simulink model "mpc_02_sim"  (R2020b)
settings: Solver=ode4  StartTime=0.0  StopTime=t_sim  FixedStep=T  RelTol=1e-3
values from neighbouring files (symbols this model uses):
  v_des = 1    [main_mpc_02.m]
  x0 = [1; 1; pi/2]    [main_mpc_02.m]
undefined symbols (not defined in the file or in its folder): mpc_ctrl_param
settings Model: Creator=vince  LastModifiedBy=vince
settings DataIOCC: ReturnWorkspaceOutputs=off

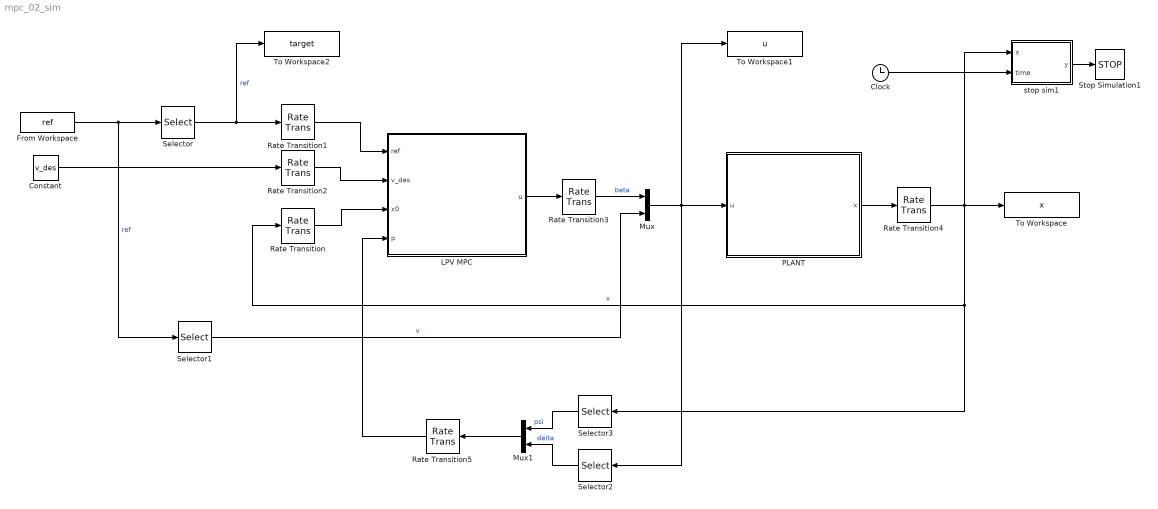
== system mpc_02_sim ==
  Clock : Clock
  Constant : Constant  Value=v_des
  From Workspace : FromWorkspace  VariableName=ref
  LPV MPC : Subsystem
  Mux : Mux  Inputs=2
  Mux1 : Mux  Inputs=2
  PLANT : Subsystem
  Rate Transition{,1..2,5} (4 alike) : RateTransition  OutPortSampleTime=mpc_ctrl_param.Ts
  Rate Transition3 : RateTransition  OutPortSampleTime=T
  Rate Transition4 : RateTransition  OutPortSampleTime=T
  Selector : Selector  InputPortWidth=4  IndexOptions=Index vector (dialog)  Indices=1:2  OutputSizes=1
  Selector1 : Selector  InputPortWidth=4  IndexOptions=Index vector (dialog)  Indices=4  OutputSizes=1
  Selector2 : Selector  InputPortWidth=2  IndexOptions=Index vector (dialog)  Indices=1  OutputSizes=1
  Selector3 : Selector  InputPortWidth=3  IndexOptions=Index vector (dialog)  Indices=3  OutputSizes=1
  Stop Simulation1 : Stop
  To Workspace : ToWorkspace  VariableName=x  SaveFormat=Timeseries  SampleTime=-1
  To Workspace1 : ToWorkspace  VariableName=u  SaveFormat=Timeseries  SampleTime=-1
  To Workspace2 : ToWorkspace  VariableName=target  SaveFormat=Timeseries  SampleTime=-1
  stop sim1 : MATLAB Function  TreatAsAtomicUnit=on
  wires:
  PLANT/1(x) -> Rate Transition4/1
  LPV MPC/1(u) -> Rate Transition3/1
  Rate Transition1/1 -> LPV MPC/1(ref)
  Rate Transition/1 -> LPV MPC/3(x0)
  Mux/1 -> To Workspace1/1, PLANT/1(u), Selector2/1
  From Workspace/1 -> Selector1/1, Selector/1  "ref"
  Selector/1 -> To Workspace2/1, Rate Transition1/1  "ref"
  Rate Transition3/1 -> Mux/1  "beta"
  Selector1/1 -> Mux/2  "v"
  Clock/1 -> stop sim1/2(time)
  stop sim1/1(y) -> Stop Simulation1/1
  Rate Transition4/1 -> stop sim1/1(x), To Workspace/1, Selector3/1, Rate Transition/1  "x"
  Mux1/1 -> Rate Transition5/1
  Rate Transition5/1 -> LPV MPC/4(p)
  Selector2/1 -> Mux1/2  "delta"
  Selector3/1 -> Mux1/1  "psi"
  Constant/1 -> Rate Transition2/1
  Rate Transition2/1 -> LPV MPC/2(v_des)

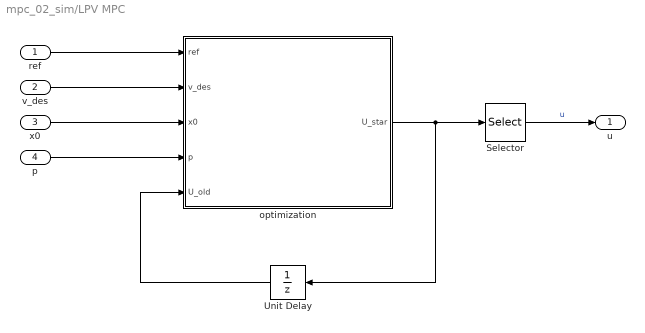
== system mpc_02_sim/LPV MPC ==
  ref : Inport
  v_des : Inport  Port=2
  x0 : Inport  Port=3
  p : Inport  Port=4
  Selector : Selector  InputPortWidth=mpc_ctrl_param.nu*mpc_ctrl_param.Nc  IndexOptions=Index vector (dialog)  Indices=1:mpc_ctrl_param.nu  OutputSizes=1
  Unit Delay : UnitDelay  InitialCondition=zeros(mpc_ctrl_param.nu*mpc_ctrl_param.Nc, 1)  SampleTime=mpc_ctrl_param.Ts  HasFrameUpgradeWarning=on
  optimization : MATLAB Function  TreatAsAtomicUnit=on
  u : Outport
  wires:
  optimization/1(U_star) -> Unit Delay/1, Selector/1
  ref/1 -> optimization/1(ref)
  x0/1 -> optimization/3(x0)
  Unit Delay/1 -> optimization/5(U_old)
  Selector/1 -> u/1  "u"
  p/1 -> optimization/4(p)
  v_des/1 -> optimization/2(v_des)

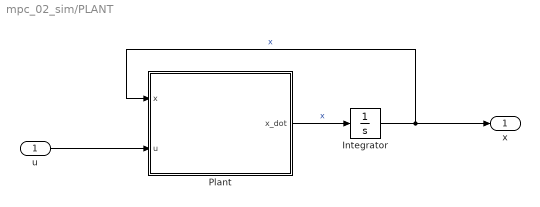
== system mpc_02_sim/PLANT ==
  u : Inport
  Integrator : Integrator  InitialCondition=x0
  Plant : MATLAB Function  TreatAsAtomicUnit=on
  x : Outport
  wires:
  u/1 -> Plant/2(u)
  Plant/1(x_dot) -> Integrator/1  "x"
  Integrator/1 -> x/1, Plant/1(x)  "x"

== matlab function mpc_02_sim/LPV MPC/optimization ==
  data: ref input; v_des input; U_star output; x0 input; p input; U_old input; mpc_ctrl_param parameter
function U_star = mpc_optimization(ref, v_des, x0, p, U_old, mpc_ctrl_param)
%% Documentation
%{

    IN: ref, x, U_old
    OUT: U*
    
    Ts = mpc_param.Ts;
    nx = mpc_param.nx;
    ny = mpc_param.ny;
    nu = mpc_param.nu;
    np = mpc_param.np;
    Np = mpc_param.Np;
    Nc = mpc_param.Nc;
    Q = mpc_param.Q;
    R = mpc_param.R;

    x_c = mpc_param.x_c
    u_c = mpc_param.u_c
    du_c = mpc_param.du_c

    Ad = pred_model.Ad;
    Bd = pred_model.Bd
    Bvd = pred_model.Bvd
    Cd = pred_model.Cd
    Dd = pred_model.Dd
    Dvd = pred_model.Dvd

    A_bar = mpc.A_bar;
    B_bar = mpc.B_bar;
    C_bar = mpc.C_bar;
    D_bar = mpc.D_bar;
    Bv_bar = mpc.Bv_bar;
    Dvd_bar = mpc.Dv_bar;
    Q_bar = mpc.Q_bar;
    R_bar = mpc.R_bar;
    X_min = mpc.X_min;
    X_max = mpc.X_max;
    U_min = mpc.U_min;
    U_max = mpc.U_max;
    dU_min = mpc.dU_min;
    dU_max = mpc.dU_max;

%}


%% Prediction model
% pred_model = bicycle_sl_position_model(mpc_ctrl_param.Ts, [x0; u0]);
pred_model = bicycle_sl_position_model(mpc_ctrl_param.Ts, v_des, p);



%% MPC QP design
mpc = mpc_design(mpc_ctrl_param, pred_model, ref);



%% Objective function
H = mpc.R_bar + mpc.D_bar'*mpc.Q_bar*mpc.D_bar;
H = (H+H')/2;
f = (mpc.C_bar*x0+mpc.L_bar-mpc.REF)'*mpc.Q_bar*(mpc.D_bar);



%% Constraints
A_ineq = [-mpc.B_bar;
          mpc.B_bar;
          -eye(mpc_ctrl_param.nu*mpc_ctrl_param.Nc);
          eye(mpc_ctrl_param.nu*mpc_ctrl_param.Nc);
          -eye(mpc_ctrl_param.nu*mpc_ctrl_param.Nc);
          eye(mpc_ctrl_param.nu*mpc_ctrl_param.Nc)];

b_ineq = [-mpc.X_min+mpc.A_bar*x0+mpc.K_bar;
          mpc.X_max-mpc.A_bar*x0-mpc.K_bar;
          -mpc.U_min;
          mpc.U_max;
          -mpc.dU_min-U_old;
          mpc.dU_max+U_old];



%% Optimization: J(u(k)) = U(k)'*H*U(k) + f'*U(k)
coder.extrinsic('quadprog');
% options = optimoptions('quadprog', 'Algorithm', 'active-set', 'Display', 'iter');

U_star = zeros(mpc_ctrl_param.nu*mpc_ctrl_param.Nc, 1);
U_star = quadprog(H, f, A_ineq, b_ineq, [], [], [], [], []);

== matlab function mpc_02_sim/PLANT/Plant ==
  data: x input; u input; x_dot output
function x_dot = mpc_pred_disc(x, u)


lr = 0.75;
psi = x(3);
beta = u(1);
v = u(2); 

%% Nonlinear model
x_dot = [v*cos(psi+beta)
    v*sin(psi+beta)
    v/lr*sin(beta)];

== matlab function mpc_02_sim/stop sim1 ==
  data: x input; y output; x_ref parameter; time input
function y = stop_sim(x, x_ref, time)

y = 0;

if (abs(x(1:2) - x_ref(1:2)) <= 1)
    y = 1;
elseif (time > 160)
    y = 1;
end
